simulink model "Tricopter_Controlled"  (R2015a)
settings: Solver=ode3  SolverMode=SingleTasking  StartTime=0.0  StopTime=inf  FixedStep=T_sim  RelTol=1e-3
values from neighbouring files (symbols this model uses):
  A_l_max_x = sqrt( (A_z_max)^2  -  g^2  )    [Run3Copter.m]
  A_l_max_y = g*tand(15)    [Run3Copter.m]
  A_z_max = Max_Thrust*3/m    [Run3Copter.m]
  Alt_0 = input(' Give the initial altitude (m): ')    [Run3Copter.m]
  B_hover_4dof = [-0.192641491537 -0.295051706147 -72.3190840892 -0.00308714144823 24.9504828653 -1.18743631629 9.87469464114e-05 6.48783896558 -0.0529805907426 -0.000387203135788 0.131620058452 2.24065603044 ... (54 elements, 6x9)]    [Effectiv_matrices.mat]
  CG_0 = [0,0,0.02]'    [SetupComplete.m]
  epsilon = 0.01    [Run3Copter.m]
  eta_23 = deg2rad(-1.3)    [Run3Copter.m]
  g = 9.81    [SetupComplete.m]
  h = 0.08    [SetupComplete.m]
  h_M = 0.064    [SetupComplete.m]
  Hover_eta_23 = deg2rad(-1.3)    [Run3Copter.m]
  Hover_throtle_1 = 0.745    [Run3Copter.m]
  Hover_throtle_23 = Hover_throtle_1/cos(Hover_eta_23)    [Run3Copter.m]
  I_BAC_0 = [ Ix,0,Ixz;0,Iy,0;Ixz,0,Iz]    [SetupComplete.m]
  Initial_Omegas = Omega_hover    [Run3Copter.m]
  Initial_Torques = Torque_hover    [Run3Copter.m]
  Ix = 0.103    [SetupComplete.m]
  Iy = 0.147    [SetupComplete.m]
  Iz = 0.237    [SetupComplete.m]
  l = 0.345    [SetupComplete.m]
  l_arm = 0.264    [SetupComplete.m]
  latitude = 52.071118    [Run3Copter.m]
  longitude = -0.627404    [Run3Copter.m]
  m = 3.51    [SetupComplete.m]
  m_0 = 2.61    [SetupComplete.m]
  m_M = 0.300    (= 0.3)    [SetupComplete.m]
  Rotation_sign = [ 1,-1,-1]    [SetupComplete.m]
  T_ctrl = 0.02    [Run3Copter.m]
  T_sim = 0.01    [Run3Copter.m]
  throtle_1 = 0*0.745    (= 0)    [Run3Copter.m]
  throtle_23 = throtle_1/cos(eta_23)    [Run3Copter.m]
  v_i0 = sqrt( 1/3*m*g/(2*rho*pi*R^2)  )    [SetupComplete.m]
undefined symbols (not defined in the file or in its folder): DOWN_0, EAST_0, Newton, NORTH_0, P_0, Q_0, R_0, Raphson, U_0, V_0, W_0
libraries: XXCopter_Control x64, simulink_extras x17, simulink x11, XXCopter x8
(part 4 of 6)

== system Tricopter_Controlled/TriCopter FCS/TriCopter FCS/Control and guidance/Inner PI Controller Quaternions/Attitude Controller ==
  AWU : Inport
  Phi_ref (rad) : Inport  Port=2
  q_ref : Inport  Port=3
  Yaw_ref (rad) : Inport  Port=4
  All_meas : Inport  Port=5
  activation_bus : Inport  Port=6
  init_cond : Inport  Port=7
  AWU1 : InportShadow
  AWU2 : InportShadow
  Build Pseudo_theta : MATLAB Function  TreatAsAtomicUnit=on
  Build Pseudo_theta1 : MATLAB Function  TreatAsAtomicUnit=on
  Bus Creator : BusCreator  Inputs=3
  Bus Creator1 : BusCreator  Inputs=3
  Bus Creator2 : BusCreator  Inputs=3
  Bus Selector : BusSelector  OutputSignals=Meas.Eulr_meas_rad,Meas.q_meas
  Bus Selector1 : BusSelector  OutputSignals=att_act
  Bus Selector2 : BusSelector  OutputSignals=att_init
  Bus Selector3 : BusSelector  OutputSignals=att_init
  Bus Selector4 : BusSelector  OutputSignals=att_init
  Mux : Mux  Inputs=3
  Ref Model and PI Controller : XXCopter_Control/Ref Model and PI Controller  delta=0  tau=2  RisingSlewLimit=deg2rad(8)  FallingSlewLimit=-deg2rad(8)  K_f=0  K_a=1  Con_way=pro  omega_n=4  xi=0.5  Z1=-30  K_b=2  f_i=0.15  f_c=1
  Ref Model and PI Controller1 : XXCopter_Control/Ref Model and PI Controller  delta=0  tau=1.5  RisingSlewLimit=deg2rad(8)  FallingSlewLimit=-deg2rad(8)  K_f=0  K_a=1  Con_way=pro  omega_n=4  xi=0.5  Z1=-30  K_b=1.2  f_i=0.1  f_c=1
  Ref Model and PI Controller2 : XXCopter_Control/Ref Model and PI Controller  delta=0  tau=1.5  RisingSlewLimit=deg2rad(8)  FallingSlewLimit=-deg2rad(8)  K_f=0  K_a=1  Con_way=pro  omega_n=4  xi=0.5  Z1=-30  K_b=1.5  f_i=0.1  f_c=1
  Retrieve quaternion : MATLAB Function  TreatAsAtomicUnit=on
  Selector : Selector  InputPortWidth=3
  Selector1 : Selector  InputPortWidth=3
  Selector2 : Selector  InputPortWidth=3  Indices=3
  Selector3 : Selector  InputPortWidth=3  Indices=2
  Selector4 : Selector  InputPortWidth=3  Indices=3
  Selector5 : Selector  InputPortWidth=3
  Selector6 : Selector  InputPortWidth=3  Indices=2
  Selector7 : Selector  InputPortWidth=3  Indices=3
  Sum : Sum  Inputs=+-|
  Sum1 : Sum  Inputs=+-|
  Sum2 : Sum  Inputs=+-|
  Terminator1 : Terminator
  Terminator2 : Terminator
  Terminator3 : Terminator
  Trigonometric Function : Trigonometry
  init_cond1 : InportShadow  Port=7
  init_cond2 : InportShadow  Port=7
  quat_dot des (rad/s) : Outport
  wires:
  Ref Model and PI Controller/4 -> Sum2/2
  Sum2/1 -> Bus Creator2/3  "Vz_err"
  Ref Model and PI Controller/3 -> Bus Creator2/2, Sum2/1  "Vz_sf"
  Ref Model and PI Controller/2 -> Bus Creator2/1  "Vz_sf_dot"
  Ref Model and PI Controller1/4 -> Sum1/2
  Sum1/1 -> Bus Creator1/3  "Vy_err"
  Ref Model and PI Controller1/3 -> Bus Creator1/2, Sum1/1  "Vy_sf"
  Ref Model and PI Controller1/2 -> Bus Creator1/1  "Vy_sf_dot"
  Ref Model and PI Controller2/4 -> Sum/2
  Bus Creator2/1 -> Terminator3/1
  Bus Creator1/1 -> Terminator1/1
  Bus Creator/1 -> Terminator2/1
  Sum/1 -> Bus Creator/3  "Vx_err"
  Ref Model and PI Controller2/3 -> Bus Creator/2, Sum/1  "Vx_sf"
  Ref Model and PI Controller2/2 -> Bus Creator/1  "Vx_sf_dot"
  Yaw_ref (rad)/1 -> Ref Model and PI Controller/1
  Selector/1 -> Ref Model and PI Controller2/2
  Bus Selector/2 -> Retrieve quaternion/2(q), Build Pseudo_theta1/1(q)  "<q_meas>"
  All_meas/1 -> Bus Selector/1
  q_ref/1 -> Build Pseudo_theta/1(q)
  Phi_ref (rad)/1 -> Ref Model and PI Controller2/1
  Retrieve quaternion/1(qdot) -> quat_dot des (rad/s)/1
  Ref Model and PI Controller2/1 -> Mux/1
  Ref Model and PI Controller/1 -> Mux/3
  Ref Model and PI Controller1/1 -> Mux/2
  Mux/1 -> Retrieve quaternion/1(Pseudoeuler_dot)
  Selector2/1 -> Ref Model and PI Controller/2
  Bus Selector/1 -> Selector2/1, Selector/1  "<Eulr_meas_rad>"
  Build Pseudo_theta1/1(Pseudo_theta) -> Ref Model and PI Controller1/2
  Build Pseudo_theta/1(Pseudo_theta) -> Ref Model and PI Controller1/1
  AWU/1 -> Selector1/1
  AWU1/1 -> Selector3/1
  AWU2/1 -> Selector4/1
  Selector3/1 -> Trigonometric Function/1
  Selector1/1 -> Ref Model and PI Controller2/4
  Trigonometric Function/1 -> Ref Model and PI Controller1/4
  Selector4/1 -> Ref Model and PI Controller/4
  activation_bus/1 -> Bus Selector1/1
  Bus Selector1/1 -> Ref Model and PI Controller/Enable, Ref Model and PI Controller1/Enable, Ref Model and PI Controller2/Enable  "<att_act>"
  init_cond/1 -> Bus Selector2/1
  Bus Selector2/1 -> Selector5/1  "<att_init>"
  Selector5/1 -> Ref Model and PI Controller2/3
  Selector6/1 -> Ref Model and PI Controller1/3
  init_cond1/1 -> Bus Selector3/1
  Bus Selector3/1 -> Selector6/1  "<att_init>"
  init_cond2/1 -> Bus Selector4/1
  Selector7/1 -> Ref Model and PI Controller/3
  Bus Selector4/1 -> Selector7/1  "<att_init>"

== system Tricopter_Controlled/TriCopter FCS/TriCopter FCS/Control and guidance/Inner PI Controller Quaternions/Body Rates Controller ==
  p_ref : Inport
  q_ref : Inport  Port=2
  r_ref : Inport  Port=3
  All_meas : Inport  Port=4
  init_cond : Inport  Port=5
  activation_bus : Inport  Port=6
  Bus Creator : BusCreator
  Bus Creator1 : BusCreator
  Bus Creator2 : BusCreator
  Bus Selector : BusSelector  OutputSignals=Meas.omega_b_meas_radps
  Bus Selector1 : BusSelector  OutputSignals=omega_b_act
  Bus Selector2 : BusSelector  OutputSignals=b_rates_init
  Bus Selector3 : BusSelector  OutputSignals=b_rates_init
  Bus Selector4 : BusSelector  OutputSignals=b_rates_init
  Mux : Mux  Inputs=3
  Ref Model and P Controller p : XXCopter_Control/Ref Model and P Controller  tau=0.7  RisingSlewLimit=4  FallingSlewLimit=-4  K_f=0.7  K_b=6
  Ref Model and P Controller q : XXCopter_Control/Ref Model and P Controller  tau=0.7  RisingSlewLimit=4  FallingSlewLimit=-4  K_f=0.7  K_b=6
  Ref Model and P Controller r : XXCopter_Control/Ref Model and P Controller  tau=1.5  RisingSlewLimit=4  FallingSlewLimit=-4  K_f=0.7  K_b=1.5
  Selector : Selector  InputPortWidth=3
  Selector1 : Selector  InputPortWidth=3  Indices=2
  Selector2 : Selector  InputPortWidth=3  Indices=3
  Selector3 : Selector  InputPortWidth=3
  Selector4 : Selector  InputPortWidth=3  Indices=2
  Selector5 : Selector  InputPortWidth=3  Indices=3
  Sum : Sum  Inputs=+-|
  Sum1 : Sum  Inputs=+-|
  Sum2 : Sum  Inputs=+-|
  Terminator1 : Terminator
  Terminator2 : Terminator
  Terminator3 : Terminator
  init_cond1 : InportShadow  Port=5
  init_cond2 : InportShadow  Port=5
  Angular acc des (rad/s^2) : Outport
  wires:
  Ref Model and P Controller r/5 -> Bus Creator2/4  "K_b_r"
  Ref Model and P Controller r/4 -> Sum2/2
  Sum2/1 -> Bus Creator2/3  "r_err"
  Ref Model and P Controller r/3 -> Bus Creator2/2, Sum2/1  "r_sf"
  Ref Model and P Controller r/2 -> Bus Creator2/1  "r_sf_dot"
  Ref Model and P Controller q/5 -> Bus Creator1/4  "K_b_q"
  Ref Model and P Controller q/4 -> Sum1/2
  Sum1/1 -> Bus Creator1/3  "q_err"
  Ref Model and P Controller q/3 -> Bus Creator1/2, Sum1/1  "q_sf"
  Ref Model and P Controller q/2 -> Bus Creator1/1  "q_sf_dot"
  Ref Model and P Controller p/5 -> Bus Creator/4  "K_b_p"
  Ref Model and P Controller p/4 -> Sum/2
  Selector2/1 -> Ref Model and P Controller r/2
  Bus Creator2/1 -> Terminator3/1
  Bus Creator1/1 -> Terminator1/1
  Bus Creator/1 -> Terminator2/1
  Sum/1 -> Bus Creator/3  "p_err"
  Ref Model and P Controller p/3 -> Bus Creator/2, Sum/1  "p_sf"
  Ref Model and P Controller p/2 -> Bus Creator/1  "p_sf_dot"
  r_ref/1 -> Ref Model and P Controller r/1
  Selector1/1 -> Ref Model and P Controller q/2
  q_ref/1 -> Ref Model and P Controller q/1
  Mux/1 -> Angular acc des (rad/s^2)/1
  p_ref/1 -> Ref Model and P Controller p/1
  Bus Selector/1 -> Selector2/1, Selector/1, Selector1/1  "<omega_b_meas_radps>"
  All_meas/1 -> Bus Selector/1
  Ref Model and P Controller r/1 -> Mux/3
  Ref Model and P Controller q/1 -> Mux/2
  Ref Model and P Controller p/1 -> Mux/1
  Selector/1 -> Ref Model and P Controller p/2
  activation_bus/1 -> Bus Selector1/1
  Bus Selector1/1 -> Ref Model and P Controller p/Enable, Ref Model and P Controller r/Enable, Ref Model and P Controller q/Enable  "<omega_b_act>"
  init_cond/1 -> Bus Selector2/1
  Bus Selector2/1 -> Selector3/1  "<b_rates_init>"
  Selector3/1 -> Ref Model and P Controller p/3
  init_cond1/1 -> Bus Selector3/1
  Bus Selector3/1 -> Selector4/1  "<b_rates_init>"
  Selector4/1 -> Ref Model and P Controller q/3
  init_cond2/1 -> Bus Selector4/1
  Bus Selector4/1 -> Selector5/1  "<b_rates_init>"
  Selector5/1 -> Ref Model and P Controller r/3

== system Tricopter_Controlled/TriCopter FCS/TriCopter FCS/Control and guidance/Inner PI Controller Quaternions/Limits in Ang accel ==
  note: Here it is assumed that at all time every prop is generating m*g/3 newtons of force . It is conservative?
  Ang Ace des : Inport
  Euler meas : Inport  Port=2
  Limis eval : MATLAB Function  TreatAsAtomicUnit=on
  Saturation Dynamic : simulink/Discontinuities/Saturation Dynamic  OutMin=[]  OutMax=[]  OutDataTypeStr=Inherit: Same as second input  OutDataType=fixdt(1, 16)  OutScaling=2^-10  DoSatur=off
  ang Ace des : Outport
  wires:
  Limis eval/1(Limit_up) -> Saturation Dynamic/1
  Limis eval/2(Limit_down) -> Saturation Dynamic/3
  Euler meas/1 -> Limis eval/2(euler_ang)
  Ang Ace des/1 -> Saturation Dynamic/2, Limis eval/1(Ang_Accel)
  Saturation Dynamic/1 -> ang Ace des/1

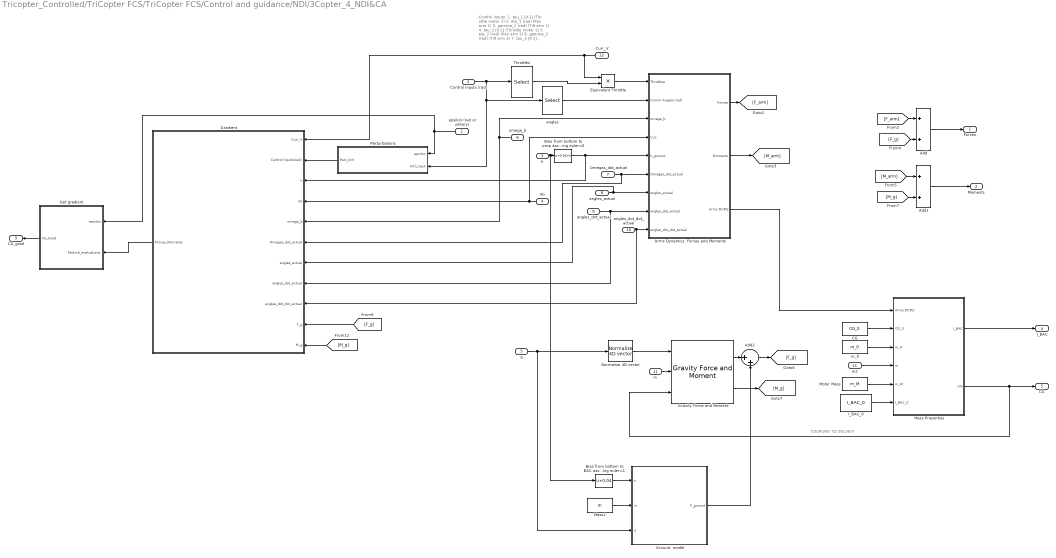
== system Tricopter_Controlled/TriCopter FCS/TriCopter FCS/Control and guidance/NDI/3Copter_4_NDI&CA ==
  note: Control inputs:
      | 1. tau_1 [0-1] (Thr ottle motor 1)
      | 2. eta_1 (rad)  (Pan arm 1)
      | 3. gamma_1 (rad)  (Tilt arm 1)
      |
      | 4. tau_2 [0-1] (Throttle motor 2)
      | 5. eta_2 (rad)  (Pan arm 2)
      | 6. gamma_2 (rad)  (Tilt arm 2)
      |
      | 7. tau_3 [0-1] (Throttle motor 3)
      | 8. eta_3 (rad)  (Pan arm  3)
      | 9. gamma_3 (rad)  (Tilt arm 3)
  note: COUPLING TO SOLVE!!!
  "epsilon (rad or unitary) " : Inport
  Control Inputs (rad) : Inport  Port=2
  h : Inport  Port=3
  Vb : Inport  Port=4
  q : Inport  Port=5
  omega_b : Inport  Port=6
  Omegas_dot_actual : Inport  Port=7
  angles_actual : Inport  Port=8
  angles_dot_actual : Inport  Port=9
  angles_dot_dot_actual : Inport  Port=10
  " m" : Inport  Port=11
  Curr_V : Inport  Port=12
  Add : Sum
  Add1 : Sum
  Add2 : Sum  Inputs=|++
  Arms Dynamics: Forces and Moments : Subsystem  TreatAsAtomicUnit=on
  Bias from bottom to BAC assuming euler=1 : Bias  Bias=0.04
  Bias from bottom to prop assuming euler=0 : Bias  Bias=0.04+h
  CG : Constant  Value=CG_0
  Equivalent Throttle : Product  Inputs=**
  Get gradient : MATLAB Function  TreatAsAtomicUnit=on
  Gradient : Subsystem  TreatAsAtomicUnit=on
  Gravity Force and Moment : XXCopter_Control/Gravity Force and Moment
  Ground  model : Subsystem  TreatAsAtomicUnit=on
  I_BAC_0 : Constant  Value=I_BAC_0
  Mass Properties : Subsystem  TreatAsAtomicUnit=on
  Mass2 : Constant  Value=m
  Motor Mass : Constant  Value=m_M
  Normalize 4D vector : XXCopter/Normalize 4D vector
  Perturbations : MATLAB Function  TreatAsAtomicUnit=on
  Throttles : Selector  IndexMode=Zero-based  InputPortWidth=9  Indices=[0,3,6]
  "angles " : Selector  IndexMode=Zero-based  InputPortWidth=9  Indices=[1,2,4,5,7,8]
  m2 : InportShadow  Port=11
  m_0 : Constant  Value=m_0
  Forces : Outport
  Moments : Outport  Port=2
  CA_grad : Outport  Port=3
  I_BAC : Outport  Port=4
  "CG " : Outport  Port=5
  wires:
  Get gradient/1(CA_Grad) -> CA_grad/1
  "epsilon (rad or unitary) "/1 -> Perturbations/1(epsilon), Get gradient/1(epsilon)
  Perturbations/1(Pert_Ctrl) -> Gradient/2("Control Inputs(rad) ")
  Gradient/1(Forces_Moments) -> Get gradient/2(Perturb_evaluations)
  Mass Properties/1(I_BAC) -> I_BAC/1
  [F_g] -> Gradient/10(F_g)
  [M_g] -> Gradient/11(M_g)
  Normalize 4D vector/1 -> Gravity Force and Moment/1
  angles_dot_actual/1 -> Arms Dynamics: Forces and Moments/8(angles_dot_actual), Gradient/8(angles_dot_actual)
  Omegas_dot_actual/1 -> Gradient/6(Omegas_dot_actual), Arms Dynamics: Forces and Moments/6(Omegas_dot_actual)
  Add1/1 -> Moments/1
  Curr_V/1 -> Gradient/1(Curr_V), Equivalent Throttle/1
  Equivalent Throttle/1 -> Arms Dynamics: Forces and Moments/1(Throttles)
  Mass Properties/2(CG) -> Gravity Force and Moment/3, "CG "/1
  Add/1 -> Forces/1
  m2/1 -> Mass Properties/4(m)
  m_0/1 -> Mass Properties/3(m_0)
  I_BAC_0/1 -> Mass Properties/6(I_BAC_0)
  Motor Mass/1 -> Mass Properties/5(m_M)
  CG/1 -> Mass Properties/2(CG_0)
  Arms Dynamics: Forces and Moments/3(Arms DCMs) -> Mass Properties/1(Arms DCMs)
  Control Inputs (rad)/1 -> Throttles/1, Perturbations/2(Ctrl_input), "angles "/1
  Throttles/1 -> Equivalent Throttle/2
  [M_g] -> Add1/2
  [M_arm] -> Add1/1
  [F_g] -> Add/2
  [F_arm] -> Add/1
  Gravity Force and Moment/2 -> [M_g]
  Arms Dynamics: Forces and Moments/2(Moments) -> [M_arm]
  Arms Dynamics: Forces and Moments/1(Forces) -> [F_arm]
  " m"/1 -> Gravity Force and Moment/2
  omega_b/1 -> Gradient/5(omega_b), Arms Dynamics: Forces and Moments/3(omega_b)
  Vb/1 -> Arms Dynamics: Forces and Moments/4(V_b), Gradient/4(Vb)
  angles_actual/1 -> Gradient/7(angles_actual), Arms Dynamics: Forces and Moments/7(angles_actual)
  "angles "/1 -> Arms Dynamics: Forces and Moments/2(Comm Angles (rad))
  angles_dot_dot_actual/1 -> Gradient/9(angles_dot_dot_actual), Arms Dynamics: Forces and Moments/9(angles_dot_dot_actual)
  Bias from bottom to prop assuming euler=0/1 -> Arms Dynamics: Forces and Moments/5(h_ground), Gradient/3(h)
  Ground  model/1(F_ground) -> Add2/2
  q/1 -> Normalize 4D vector/1, Ground  model/3(q)
  Mass2/1 -> Ground  model/2(m)
  Bias from bottom to BAC assuming euler=1/1 -> Ground  model/1(h)
  h/1 -> Bias from bottom to prop assuming euler=0/1, Bias from bottom to BAC assuming euler=1/1
  Gravity Force and Moment/1 -> Add2/1
  Add2/1 -> [F_g]

== system Tricopter_Controlled/TriCopter FCS/TriCopter FCS/Control and guidance/Otter Overactuated P Controller/Position Controller ==
  AWU : Inport
  X_e_x_ref : Inport  Port=2
  X_e_y_ref : Inport  Port=3
  X_e_z_ref : Inport  Port=4
  activation_bus : Inport  Port=5
  All_meas : Inport  Port=6
  init_cond : Inport  Port=7
  AWU1 : InportShadow
  AWU2 : InportShadow
  Bus Creator : BusCreator  Inputs=3
  Bus Creator1 : BusCreator  Inputs=3
  Bus Creator2 : BusCreator  Inputs=3
  Bus Selector : BusSelector  OutputSignals=Meas.Pos_meas_m
  Bus Selector1 : BusSelector  OutputSignals=pos_xy_init
  Bus Selector2 : BusSelector  OutputSignals=pos_xy_act
  Bus Selector3 : BusSelector  OutputSignals=alt_init
  Bus Selector4 : BusSelector  OutputSignals=alt_act
  Mux : Mux  Inputs=3
  Ref Model and PI Controller : XXCopter_Control/Ref Model and PI Controller  delta=0  tau=3  RisingSlewLimit=4  FallingSlewLimit=-4  K_f=0  K_a=1  Con_way=pro  omega_n=4  xi=0.5  Z1=-30  K_b=1.2  f_i=0.07  f_c=1
  Ref Model and PI Controller1 : XXCopter_Control/Ref Model and PI Controller  delta=0  tau=5  RisingSlewLimit=4  FallingSlewLimit=-4  K_f=0  K_a=1  Con_way=pro  omega_n=4  xi=0.5  Z1=-30  K_b=1  f_i=0.07  f_c=1
  Ref Model and PI Controller3 : XXCopter_Control/Ref Model and PI Controller  delta=0  tau=5  RisingSlewLimit=4  FallingSlewLimit=-4  K_f=0  K_a=1  Con_way=pro  omega_n=4  xi=0.5  Z1=-30  K_b=1  f_i=0.07  f_c=1
  Selector : Selector  InputPortWidth=3
  Selector1 : Selector  InputPortWidth=3  Indices=2
  Selector2 : Selector  InputPortWidth=3  Indices=3
  Selector3 : Selector  InputPortWidth=3
  Selector4 : Selector  InputPortWidth=3  Indices=2
  Selector5 : Selector  InputPortWidth=3  Indices=3
  Selector6 : Selector  InputPortWidth=2
  Selector7 : Selector  InputPortWidth=2  Indices=2
  Sum : Sum  Inputs=+-|
  Sum1 : Sum  Inputs=+-|
  Sum2 : Sum  Inputs=+-|
  Terminator1 : Terminator
  Terminator2 : Terminator
  Terminator3 : Terminator
  Ve des (m/s) : Outport
  wires:
  All_meas/1 -> Bus Selector/1
  Bus Selector/1 -> Selector/1, Selector1/1, Selector2/1  "<Pos_meas_m>"
  X_e_x_ref/1 -> Ref Model and PI Controller3/1
  Ref Model and PI Controller3/1 -> Mux/1
  Mux/1 -> Ve des (m/s)/1
  X_e_y_ref/1 -> Ref Model and PI Controller1/1
  X_e_z_ref/1 -> Ref Model and PI Controller/1
  Ref Model and PI Controller1/1 -> Mux/2
  Ref Model and PI Controller/1 -> Mux/3
  Ref Model and PI Controller3/2 -> Bus Creator/1  "X_ex_sf_dot"
  Ref Model and PI Controller3/3 -> Bus Creator/2, Sum/1  "X_ex_sf"
  Sum/1 -> Bus Creator/3  "X_ex_err"
  Bus Creator/1 -> Terminator2/1
  Bus Creator1/1 -> Terminator1/1
  Bus Creator2/1 -> Terminator3/1
  Ref Model and PI Controller3/4 -> Sum/2
  Ref Model and PI Controller1/2 -> Bus Creator1/1  "X_ey_sf_dot"
  Ref Model and PI Controller1/3 -> Sum1/1, Bus Creator1/2  "X_e_y_sf"
  Sum1/1 -> Bus Creator1/3  "X_ey_err"
  Ref Model and PI Controller1/4 -> Sum1/2
  Ref Model and PI Controller/2 -> Bus Creator2/1  "X_ez_sf_dot"
  Ref Model and PI Controller/3 -> Sum2/1, Bus Creator2/2  "X_ez_sf"
  Sum2/1 -> Bus Creator2/3  "X_ez_err"
  Ref Model and PI Controller/4 -> Sum2/2
  AWU/1 -> Selector3/1
  AWU1/1 -> Selector4/1
  AWU2/1 -> Selector5/1
  Selector3/1 -> Ref Model and PI Controller3/4
  Selector4/1 -> Ref Model and PI Controller1/4
  Selector5/1 -> Ref Model and PI Controller/4
  Selector2/1 -> Ref Model and PI Controller/2
  Selector1/1 -> Ref Model and PI Controller1/2
  Selector/1 -> Ref Model and PI Controller3/2
  init_cond/1 -> Bus Selector1/1, Bus Selector3/1
  activation_bus/1 -> Bus Selector4/1, Bus Selector2/1
  Bus Selector2/1 -> Ref Model and PI Controller1/Enable, Ref Model and PI Controller3/Enable  "<pos_xy_act>"
  Bus Selector1/1 -> Selector7/1, Selector6/1  "<pos_xy_init>"
  Selector6/1 -> Ref Model and PI Controller3/3
  Selector7/1 -> Ref Model and PI Controller1/3
  Bus Selector3/1 -> Ref Model and PI Controller/3  "<alt_init>"
  Bus Selector4/1 -> Ref Model and PI Controller/Enable  "<alt_act>"

== system Tricopter_Controlled/TriCopter FCS/TriCopter FCS/Control and guidance/Otter Overactuated P Controller/Velocity Controller ==
  Vyaw_x_ref : Inport
  Vyaw_y_ref : Inport  Port=2
  Vyaw_z_ref : Inport  Port=3
  V_yaw_meas : Inport  Port=4
  activation_bus : Inport  Port=5
  Init_cond : Inport  Port=6
  Bus Creator : BusCreator
  Bus Creator1 : BusCreator
  Bus Creator2 : BusCreator
  Bus Selector1 : BusSelector  OutputSignals=vel_yaw_z_act
  Bus Selector2 : BusSelector  OutputSignals=vel_yaw_xy_act
  Bus Selector3 : BusSelector  OutputSignals=vel_yaw_xy_init
  Bus Selector4 : BusSelector  OutputSignals=vel_yaw_z_init
  Mux : Mux  Inputs=3
  Ref Model and P Controller p : XXCopter_Control/Ref Model and P Controller  tau=2  RisingSlewLimit=1  FallingSlewLimit=-1  K_f=0.5  K_b=1
  Ref Model and P Controller q : XXCopter_Control/Ref Model and P Controller  tau=2  RisingSlewLimit=1  FallingSlewLimit=-1  K_f=0.5  K_b=1
  Ref Model and P Controller r : XXCopter_Control/Ref Model and P Controller  tau=1  RisingSlewLimit=1  FallingSlewLimit=-1  K_f=0.4  K_b=8
  Selector : Selector  InputPortWidth=3
  Selector1 : Selector  InputPortWidth=3  Indices=2
  Selector2 : Selector  InputPortWidth=3  Indices=3
  Selector3 : Selector  InputPortWidth=2
  Selector4 : Selector  InputPortWidth=2  Indices=2
  Sum : Sum  Inputs=+-|
  Sum1 : Sum  Inputs=+-|
  Sum2 : Sum  Inputs=+-|
  Terminator1 : Terminator
  Terminator2 : Terminator
  Terminator3 : Terminator
  Acc_yaw des (m/s) : Outport
  wires:
  Ref Model and P Controller r/5 -> Bus Creator2/4  "K_b_Ve_z"
  Ref Model and P Controller r/4 -> Sum2/2
  Sum2/1 -> Bus Creator2/3  "Vez_err"
  Ref Model and P Controller r/3 -> Bus Creator2/2, Sum2/1  "Vez_sf"
  Ref Model and P Controller r/2 -> Bus Creator2/1  "Vez_sf_dot"
  Ref Model and P Controller q/5 -> Bus Creator1/4  "K_b_Vey"
  Ref Model and P Controller q/4 -> Sum1/2
  Sum1/1 -> Bus Creator1/3  "Vey_err"
  Ref Model and P Controller q/3 -> Bus Creator1/2, Sum1/1  "Ve_y_sf"
  Ref Model and P Controller q/2 -> Bus Creator1/1  "Vey_sf_dot"
  Ref Model and P Controller p/5 -> Bus Creator/4  "K_b_Vex"
  Ref Model and P Controller p/4 -> Sum/2
  Selector2/1 -> Ref Model and P Controller r/2
  Bus Creator2/1 -> Terminator3/1
  Bus Creator1/1 -> Terminator1/1
  Bus Creator/1 -> Terminator2/1
  Sum/1 -> Bus Creator/3  "Vex_err"
  Ref Model and P Controller p/3 -> Bus Creator/2, Sum/1  "Vex_sf"
  Ref Model and P Controller p/2 -> Bus Creator/1  "Vex_sf_dot"
  Ref Model and P Controller r/1 -> Mux/3
  Ref Model and P Controller q/1 -> Mux/2
  Vyaw_z_ref/1 -> Ref Model and P Controller r/1
  Selector1/1 -> Ref Model and P Controller q/2
  Vyaw_y_ref/1 -> Ref Model and P Controller q/1
  Mux/1 -> Acc_yaw des (m/s)/1
  Ref Model and P Controller p/1 -> Mux/1
  Vyaw_x_ref/1 -> Ref Model and P Controller p/1
  V_yaw_meas/1 -> Selector1/1, Selector/1, Selector2/1
  Selector/1 -> Ref Model and P Controller p/2
  activation_bus/1 -> Bus Selector1/1, Bus Selector2/1
  Bus Selector2/1 -> Ref Model and P Controller q/Enable, Ref Model and P Controller p/Enable  "<vel_yaw_xy_act>"
  Bus Selector1/1 -> Ref Model and P Controller r/Enable  "<vel_yaw_z_act>"
  Init_cond/1 -> Bus Selector4/1, Bus Selector3/1
  Bus Selector3/1 -> Selector3/1, Selector4/1  "<vel_yaw_xy_init>"
  Selector3/1 -> Ref Model and P Controller p/3
  Selector4/1 -> Ref Model and P Controller q/3
  Bus Selector4/1 -> Ref Model and P Controller r/3  "<vel_yaw_z_init>"

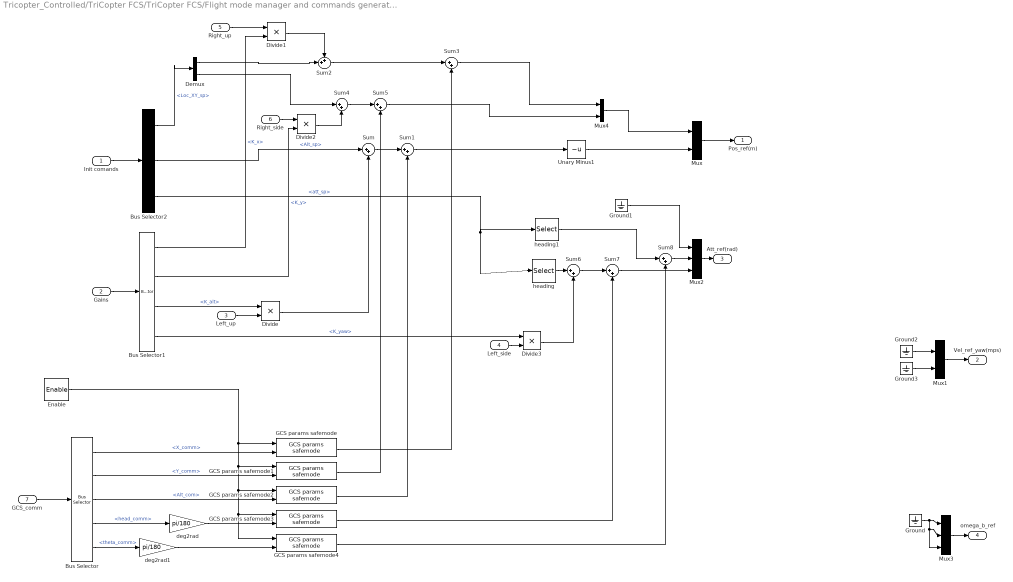
== system Tricopter_Controlled/TriCopter FCS/TriCopter FCS/Flight mode manager and commands generator/Commands generator/Full auto ==
  Init comands : Inport
  Gains : Inport  Port=2
  Left_up : Inport  Port=3
  Left_side : Inport  Port=4
  Right_up : Inport  Port=5
  Right_side : Inport  Port=6
  GCS_comm : Inport  Port=7
  Enable : EnablePort  StatesWhenEnabling=reset  ShowOutputPort=on
  Bus Selector : BusSelector  OutputSignals=X_comm,Y_comm,Alt_com,head_comm,theta_comm
  Bus Selector1 : BusSelector  OutputSignals=K_x,K_y,K_alt,K_yaw
  Bus Selector2 : BusSelector  OutputSignals=Loc_XY_sp,Alt_sp,att_sp
  Demux : Demux  Outputs=2
  Divide{,1..3} (4 alike) : Product  Inputs=**
  GCS params safemode{,1..4} (5 alike) : XXCopter_Control/GCS params safemode
  Ground{,1..3} (4 alike) : Ground
  Mux : Mux  Inputs=[2,1]
  Mux1 : Mux  Inputs=[2,1]
  Mux2 : Mux  Inputs=3
  Mux3 : Mux  Inputs=3
  Mux4 : Mux  Inputs=2
  Sum{,1,3..8} (8 alike) : Sum  Inputs=|++
  Sum2 : Sum  Inputs=++|
  Unary Minus1 : UnaryMinus
  deg2rad : Gain  Gain=pi/180
  deg2rad1 : Gain  Gain=pi/180
  heading : Selector  InputPortWidth=3  Indices=3
  heading1 : Selector  InputPortWidth=3  Indices=2
  Pos_ref(m) : Outport
  Vel_ref_yaw(mps) : Outport  Port=2
  Att_ref(rad) : Outport  Port=3
  omega_b_ref : Outport  Port=4
  wires:
  Bus Selector2/2 -> Sum/1  "<Alt_sp>"
  Divide/1 -> Sum/2
  Sum/1 -> Sum1/1
  GCS params safemode2/1 -> Sum1/2
  Sum1/1 -> Unary Minus1/1
  GCS_comm/1 -> Bus Selector/1
  Bus Selector/1 -> GCS params safemode/2  "<X_comm>"
  Bus Selector/2 -> GCS params safemode1/2  "<Y_comm>"
  Bus Selector/3 -> GCS params safemode2/2  "<Alt_com>"
  Bus Selector/4 -> deg2rad/1  "<head_comm>"
  Mux1/1 -> Vel_ref_yaw(mps)/1
  Mux/1 -> Pos_ref(m)/1
  Mux2/1 -> Att_ref(rad)/1
  Unary Minus1/1 -> Mux/2
  Ground/1 -> Mux3/3, Mux3/2, Mux3/1
  Ground1/1 -> Mux2/1
  Ground2/1 -> Mux1/1
  Ground3/1 -> Mux1/2
  Mux4/1 -> Mux/1
  Mux3/1 -> omega_b_ref/1
  Gains/1 -> Bus Selector1/1
  Init comands/1 -> Bus Selector2/1
  Bus Selector1/3 -> Divide/1  "<K_alt>"
  Left_up/1 -> Divide/2
  Bus Selector2/1 -> Demux/1  "<Loc_XY_sp>"
  Sum2/1 -> Sum3/1
  Sum3/1 -> Mux4/1
  GCS params safemode/1 -> Sum3/2
  Demux/1 -> Sum2/2
  Right_up/1 -> Divide1/1
  Bus Selector1/1 -> Divide1/2  "<K_x>"
  Divide1/1 -> Sum2/1
  Sum4/1 -> Sum5/1
  GCS params safemode1/1 -> Sum5/2
  Sum5/1 -> Mux4/2
  Divide2/1 -> Sum4/2
  Demux/2 -> Sum4/1
  Right_side/1 -> Divide2/1
  Bus Selector1/2 -> Divide2/2  "<K_y>"
  Sum6/1 -> Sum7/1
  Sum7/1 -> Mux2/3
  GCS params safemode3/1 -> Sum7/2
  heading/1 -> Sum6/1
  Bus Selector2/3 -> heading1/1, heading/1  "<att_sp>"
  Bus Selector1/4 -> Divide3/1  "<K_yaw>"
  Left_side/1 -> Divide3/2
  Divide3/1 -> Sum6/2
  Bus Selector/5 -> deg2rad1/1  "<theta_comm>"
  GCS params safemode4/1 -> Sum8/2
  heading1/1 -> Sum8/1
  Sum8/1 -> Mux2/2
  deg2rad/1 -> GCS params safemode3/2
  deg2rad1/1 -> GCS params safemode4/2
  Enable/1 -> GCS params safemode4/1, GCS params safemode3/1, GCS params safemode2/1, GCS params safemode1/1, GCS params safemode/1

== system Tricopter_Controlled/TriCopter FCS/TriCopter FCS/Flight mode manager and commands generator/Commands generator/Home ==
  Init comands : Inport
  Gains : Inport  Port=2
  Left_up : Inport  Port=3
  Left_side : Inport  Port=4
  Right_up : Inport  Port=5
  Right_side : Inport  Port=6
  GCS_comm : Inport  Port=7
  Enable : EnablePort  StatesWhenEnabling=reset
  Bus Selector2 : BusSelector  OutputSignals=Loc_XY_sp,Alt_sp,att_sp
  Ground{,1..3} (4 alike) : Ground
  Mux : Mux  Inputs=[2,1]
  Mux1 : Mux  Inputs=[2,1]
  Mux2 : Mux  Inputs=3
  Selector : Selector  InputPortWidth=3  Indices=3
  Terminator{,1..5} (6 alike) : Terminator
  Unary Minus : UnaryMinus
  Pos_ref(m) : Outport
  Vel_ref_yaw(mps) : Outport  Port=2
  Att_ref(rad) : Outport  Port=3
  omega_b_ref : Outport  Port=4
  wires:
  Mux1/1 -> Vel_ref_yaw(mps)/1
  Mux2/1 -> Att_ref(rad)/1
  Ground1/1 -> Mux2/2, Mux2/1
  Ground2/1 -> Mux1/1
  Ground3/1 -> Mux1/2
  Mux/1 -> Pos_ref(m)/1
  Ground/1 -> omega_b_ref/1
  Gains/1 -> Terminator/1
  Right_up/1 -> Terminator1/1
  Left_up/1 -> Terminator2/1
  Left_side/1 -> Terminator3/1
  Right_side/1 -> Terminator4/1
  GCS_comm/1 -> Terminator5/1
  Init comands/1 -> Bus Selector2/1
  Bus Selector2/1 -> Mux/1  "<Loc_XY_sp>"
  Bus Selector2/2 -> Unary Minus/1  "<Alt_sp>"
  Unary Minus/1 -> Mux/2
  Selector/1 -> Mux2/3
  Bus Selector2/3 -> Selector/1  "<att_sp>"

== system Tricopter_Controlled/TriCopter FCS/TriCopter FCS/Flight mode manager and commands generator/Commands generator/Land  ==
  Init comands : Inport
  Gains : Inport  Port=2
  Left_up : Inport  Port=3
  Left_side : Inport  Port=4
  Right_up : Inport  Port=5
  Right_side : Inport  Port=6
  GCS_comm : Inport  Port=7
  Enable : EnablePort  StatesWhenEnabling=reset
  Bus Selector2 : BusSelector  OutputSignals=Loc_XY_sp,Alt_sp,att_sp
  Ground{,1..3} (4 alike) : Ground
  Mux : Mux  Inputs=[2,1]
  Mux1 : Mux  Inputs=[2,1]
  Mux2 : Mux  Inputs=3
  Selector : Selector  InputPortWidth=3  Indices=3
  Terminator{,1..5} (6 alike) : Terminator
  Unary Minus : UnaryMinus
  Pos_ref(m) : Outport
  Vel_ref_yaw(mps) : Outport  Port=2
  Att_ref(rad) : Outport  Port=3
  omega_b_ref : Outport  Port=4
  wires:
  Mux1/1 -> Vel_ref_yaw(mps)/1
  Mux2/1 -> Att_ref(rad)/1
  Ground/1 -> omega_b_ref/1
  Ground1/1 -> Mux2/2, Mux2/1
  Ground2/1 -> Mux1/1
  Ground3/1 -> Mux1/2
  Mux/1 -> Pos_ref(m)/1
  Gains/1 -> Terminator/1
  Right_up/1 -> Terminator1/1
  Left_up/1 -> Terminator2/1
  Left_side/1 -> Terminator3/1
  Right_side/1 -> Terminator4/1
  GCS_comm/1 -> Terminator5/1
  Init comands/1 -> Bus Selector2/1
  Bus Selector2/1 -> Mux/1  "<Loc_XY_sp>"
  Bus Selector2/2 -> Unary Minus/1  "<Alt_sp>"
  Unary Minus/1 -> Mux/2
  Selector/1 -> Mux2/3
  Bus Selector2/3 -> Selector/1  "<att_sp>"

== system Tricopter_Controlled/TriCopter FCS/TriCopter FCS/Flight mode manager and commands generator/Commands generator/Man_ctrl ==
  Init comands : Inport
  Gains : Inport  Port=2
  Left_up : Inport  Port=3
  Left_side : Inport  Port=4
  Right_up : Inport  Port=5
  Right_side : Inport  Port=6
  GCS_comm : Inport  Port=7
  Enable : EnablePort  StatesWhenEnabling=reset
  Bus Selector1 : BusSelector  OutputSignals=K_vz,K_p,K_q,K_r
  Divide{1..4} (4 alike) : Product  Inputs=**
  Ground{1..2,4..5} (4 alike) : Ground
  Mux : Mux  Inputs=[2,1]
  Mux1 : Mux  Inputs=[2,1]
  Mux2 : Mux  Inputs=3
  Mux3 : Mux  Inputs=3
  Terminator : Terminator
  Terminator1 : Terminator
  Unary Minus : UnaryMinus
  Unary Minus1 : UnaryMinus
  Pos_ref(m) : Outport
  Vel_ref_yaw(mps) : Outport  Port=2
  Att_ref(rad) : Outport  Port=3
  omega_b_ref : Outport  Port=4
  wires:
  Mux1/1 -> Vel_ref_yaw(mps)/1
  Mux2/1 -> Att_ref(rad)/1
  Ground5/1 -> Mux/2
  Ground1/1 -> Mux2/3, Mux2/2, Mux2/1
  Ground2/1 -> Mux1/1
  Unary Minus1/1 -> Mux1/2
  Mux/1 -> Pos_ref(m)/1
  Mux3/1 -> omega_b_ref/1
  GCS_comm/1 -> Terminator/1
  Init comands/1 -> Terminator1/1
  Gains/1 -> Bus Selector1/1
  Bus Selector1/1 -> Divide1/2  "<K_vz>"
  Left_up/1 -> Divide1/1
  Ground4/1 -> Mux/1
  Bus Selector1/2 -> Divide2/1  "<K_p>"
  Right_side/1 -> Divide2/2
  Bus Selector1/3 -> Divide3/1  "<K_q>"
  Right_up/1 -> Divide3/2
  Bus Selector1/4 -> Divide4/1  "<K_r>"
  Left_side/1 -> Divide4/2
  Divide3/1 -> Unary Minus/1
  Divide2/1 -> Mux3/1
  Unary Minus/1 -> Mux3/2
  Divide4/1 -> Mux3/3
  Divide1/1 -> Unary Minus1/1

== system Tricopter_Controlled/TriCopter FCS/TriCopter FCS/Flight mode manager and commands generator/Commands generator/Off//Ready ==
  Init comands : Inport
  Gains : Inport  Port=2
  Left_up : Inport  Port=3
  Left_side : Inport  Port=4
  Right_up : Inport  Port=5
  Right_side : Inport  Port=6
  GCS_comm : Inport  Port=7
  Enable : EnablePort  StatesWhenEnabling=reset
  Ground{,1..3} (4 alike) : Ground
  Terminator{,1..5} (6 alike) : Terminator
  Pos_ref(m) : Outport
  Vel_ref_yaw(mps) : Outport  Port=2
  Att_ref(rad) : Outport  Port=3
  omega_b_ref : Outport  Port=4
  wires:
  Gains/1 -> Terminator/1
  Right_up/1 -> Terminator1/1
  Left_up/1 -> Terminator2/1
  Left_side/1 -> Terminator3/1
  Right_side/1 -> Terminator4/1
  GCS_comm/1 -> Terminator5/1
  Ground/1 -> Pos_ref(m)/1
  Ground1/1 -> Att_ref(rad)/1
  Ground2/1 -> Vel_ref_yaw(mps)/1
  Ground3/1 -> omega_b_ref/1

== system Tricopter_Controlled/TriCopter FCS/TriCopter FCS/Flight mode manager and commands generator/Commands generator/Stab ==
  Init comands : Inport
  Gains : Inport  Port=2
  Left_up : Inport  Port=3
  Left_side : Inport  Port=4
  Right_up : Inport  Port=5
  Right_side : Inport  Port=6
  GCS_comm : Inport  Port=7
  Enable : EnablePort  StatesWhenEnabling=reset  ShowOutputPort=on
  Bus Selector : BusSelector  OutputSignals=Vz_yaw_comm,head_comm
  Bus Selector1 : BusSelector  OutputSignals=K_vz,K_phi,K_theta,K_yaw
  Bus Selector2 : BusSelector  OutputSignals=Vel_yaw_z_sp,att_sp
  Divide{1..4} (4 alike) : Product  Inputs=**
  GCS params safemode2 : XXCopter_Control/GCS params safemode
  GCS params safemode3 : XXCopter_Control/GCS params safemode
  Ground{,2..4} (4 alike) : Ground
  Mux : Mux  Inputs=[2,1]
  Mux1 : Mux  Inputs=[2,1]
  Mux2 : Mux  Inputs=3
  Selector : Selector  InputPortWidth=3  Indices=3
  Sum{3,6,8..9} (4 alike) : Sum  Inputs=|++
  Unary Minus : UnaryMinus
  Unary Minus1 : UnaryMinus
  deg2rad1 : Gain  Gain=pi/180
  Pos_ref(m) : Outport
  Vel_ref_yaw(mps) : Outport  Port=2
  Att_ref(rad) : Outport  Port=3
  omega_b_ref : Outport  Port=4
  wires:
  Mux1/1 -> Vel_ref_yaw(mps)/1
  Mux2/1 -> Att_ref(rad)/1
  Mux/1 -> Pos_ref(m)/1
  Ground/1 -> omega_b_ref/1
  GCS_comm/1 -> Bus Selector/1
  Bus Selector/1 -> GCS params safemode2/2  "<Vz_yaw_comm>"
  Bus Selector/2 -> deg2rad1/1  "<head_comm>"
  deg2rad1/1 -> GCS params safemode3/2
  Bus Selector2/1 -> Sum3/1  "<Vel_yaw_z_sp>"
  Gains/1 -> Bus Selector1/1
  Init comands/1 -> Bus Selector2/1
  Sum3/1 -> Sum6/1
  Divide3/1 -> Sum3/2
  Left_up/1 -> Divide3/2
  Ground4/1 -> Mux/1
  GCS params safemode2/1 -> Sum6/2
  Sum6/1 -> Unary Minus/1
  Right_up/1 -> Divide1/1
  Right_side/1 -> Divide2/1
  Sum8/1 -> Sum9/1
  Selector/1 -> Sum8/1
  Bus Selector2/2 -> Selector/1  "<att_sp>"
  Left_side/1 -> Divide4/2
  Divide4/1 -> Sum8/2
  Sum9/1 -> Mux2/3
  GCS params safemode3/1 -> Sum9/2
  Ground2/1 -> Mux1/1
  Unary Minus/1 -> Mux1/2
  Bus Selector1/1 -> Divide3/1  "<K_vz>"
  Bus Selector1/4 -> Divide4/1  "<K_yaw>"
  Bus Selector1/2 -> Divide2/2  "<K_phi>"
  Bus Selector1/3 -> Divide1/2  "<K_theta>"
  Enable/1 -> GCS params safemode3/1, GCS params safemode2/1
  Ground3/1 -> Mux/2
  Divide2/1 -> Mux2/1
  Divide1/1 -> Unary Minus1/1
  Unary Minus1/1 -> Mux2/2

== system Tricopter_Controlled/TriCopter FCS/TriCopter FCS/Flight mode manager and commands generator/Commands generator/Take off ==
  Init comands : Inport
  Gains : Inport  Port=2
  Left_up : Inport  Port=3
  Left_side : Inport  Port=4
  Right_up : Inport  Port=5
  Right_side : Inport  Port=6
  GCS_comm : Inport  Port=7
  Enable : EnablePort  StatesWhenEnabling=reset  ShowOutputPort=on
  Bus Selector : BusSelector  OutputSignals=K_alt
  Bus Selector1 : BusSelector  OutputSignals=Alt_sp
  Bus Selector2 : BusSelector  OutputSignals=Alt_com
  Divide : Product  Inputs=**
  GCS params safemode : XXCopter_Control/GCS params safemode
  Ground{,1..4} (5 alike) : Ground
  Mux : Mux  Inputs=[2,1]
  Mux1 : Mux  Inputs=[2,1]
  Mux2 : Mux  Inputs=3
  Sum : Sum  Inputs=|++
  Sum1 : Sum  Inputs=|++
  Terminator : Terminator
  Terminator1 : Terminator
  Terminator2 : Terminator
  Unary Minus : UnaryMinus
  Pos_ref(m) : Outport
  Vel_ref_yaw(mps) : Outport  Port=2
  Att_ref(rad) : Outport  Port=3
  omega_b_ref : Outport  Port=4
  wires:
  Mux1/1 -> Vel_ref_yaw(mps)/1
  Mux/1 -> Pos_ref(m)/1
  Mux2/1 -> Att_ref(rad)/1
  Gains/1 -> Bus Selector/1
  Init comands/1 -> Bus Selector1/1
  Unary Minus/1 -> Mux/2
  GCS_comm/1 -> Bus Selector2/1
  Bus Selector1/1 -> Sum/1  "<Alt_sp>"
  Bus Selector/1 -> Divide/1  "<K_alt>"
  Left_up/1 -> Divide/2
  Divide/1 -> Sum/2
  Sum/1 -> Sum1/1
  GCS params safemode/1 -> Sum1/2
  Sum1/1 -> Unary Minus/1
  Right_up/1 -> Terminator/1
  Left_side/1 -> Terminator1/1
  Right_side/1 -> Terminator2/1
  Ground/1 -> omega_b_ref/1
  Ground1/1 -> Mux2/3, Mux2/2, Mux2/1
  Ground2/1 -> Mux1/1
  Ground3/1 -> Mux1/2
  Ground4/1 -> Mux/1
  Enable/1 -> GCS params safemode/1
  Bus Selector2/1 -> GCS params safemode/2  "<Alt_com>"

== system Tricopter_Controlled/TriCopter FCS/TriCopter FCS/Flight mode manager and commands generator/Commands generator/Vel_height_auto ==
  Init comands : Inport
  Gains : Inport  Port=2
  Left_up : Inport  Port=3
  Left_side : Inport  Port=4
  Right_up : Inport  Port=5
  Right_side : Inport  Port=6
  GCS_comm : Inport  Port=7
  Enable : EnablePort  StatesWhenEnabling=reset  ShowOutputPort=on
  Bus Selector : BusSelector  OutputSignals=Vx_yaw_comm,Vy_yaw_comm,Alt_com,head_comm,theta_comm
  Bus Selector1 : BusSelector  OutputSignals=K_vx,K_vy,K_alt,K_yaw
  Bus Selector2 : BusSelector  OutputSignals=Vel_yaw_xy_sp,Alt_sp,att_sp
  Demux : Demux  Outputs=2
  Divide{1..4} (4 alike) : Product  Inputs=**
  GCS params safemode{,1..4} (5 alike) : XXCopter_Control/GCS params safemode
  Ground{,1..3} (4 alike) : Ground
  Mux : Mux  Inputs=[2,1]
  Mux1 : Mux  Inputs=[2,1]
  Mux2 : Mux  Inputs=3
  Mux4 : Mux  Inputs=2
  Selector : Selector  InputPortWidth=3  Indices=3
  Selector1 : Selector  InputPortWidth=3  Indices=2
  Sum1 : Sum  Inputs=++|
  Sum{2..9} (8 alike) : Sum  Inputs=|++
  Unary Minus : UnaryMinus
  deg2rad1 : Gain  Gain=pi/180
  deg2rad2 : Gain  Gain=pi/180
  Pos_ref(m) : Outport
  Vel_ref_yaw(mps) : Outport  Port=2
  Att_ref(rad) : Outport  Port=3
  omega_b_ref : Outport  Port=4
  wires:
  Mux1/1 -> Vel_ref_yaw(mps)/1
  Mux2/1 -> Att_ref(rad)/1
  Unary Minus/1 -> Mux/2
  Ground1/1 -> Mux2/1
  Mux4/1 -> Mux1/1
  Ground3/1 -> Mux1/2
  Ground/1 -> omega_b_ref/1
  Mux/1 -> Pos_ref(m)/1
  Gains/1 -> Bus Selector1/1
  Init comands/1 -> Bus Selector2/1
  GCS_comm/1 -> Bus Selector/1
  Sum4/1 -> Sum5/1
  Divide2/1 -> Sum4/2
  Bus Selector2/2 -> Sum4/1  "<Alt_sp>"
  Bus Selector2/1 -> Demux/1  "<Vel_yaw_xy_sp>"
  Sum1/1 -> Sum2/1
  Demux/1 -> Sum1/2
  Right_up/1 -> Divide1/1
  Divide1/1 -> Sum1/1
  Bus Selector1/1 -> Divide1/2  "<K_vx>"
  Bus Selector/1 -> GCS params safemode/2  "<Vx_yaw_comm>"
  GCS params safemode/1 -> Sum2/2
  Bus Selector/2 -> GCS params safemode1/2  "<Vy_yaw_comm>"
  Bus Selector/3 -> GCS params safemode2/2  "<Alt_com>"
  Bus Selector/4 -> deg2rad1/1  "<head_comm>"
  Bus Selector/5 -> deg2rad2/1  "<theta_comm>"
  GCS params safemode2/1 -> Sum5/2
  Sum5/1 -> Unary Minus/1
  Bus Selector1/3 -> Divide2/2  "<K_alt>"
  Left_up/1 -> Divide2/1
  Sum3/1 -> Sum6/1
  Divide3/1 -> Sum3/2
  Right_side/1 -> Divide3/1
  Bus Selector1/2 -> Divide3/2  "<K_vy>"
  Demux/2 -> Sum3/1
  Sum2/1 -> Mux4/1
  Sum6/1 -> Mux4/2
  GCS params safemode1/1 -> Sum6/2
  Sum7/1 -> Sum8/1
  Selector/1 -> Sum7/1
  Left_side/1 -> Divide4/2
  Bus Selector2/3 -> Selector/1, Selector1/1  "<att_sp>"
  Bus Selector1/4 -> Divide4/1  "<K_yaw>"
  Sum8/1 -> Mux2/3
  Selector1/1 -> Sum9/1
  Sum9/1 -> Mux2/2
  Divide4/1 -> Sum7/2
  GCS params safemode3/1 -> Sum8/2
  GCS params safemode4/1 -> Sum9/2
  Ground2/1 -> Mux/1
  deg2rad1/1 -> GCS params safemode3/2
  deg2rad2/1 -> GCS params safemode4/2
  Enable/1 -> GCS params safemode4/1, GCS params safemode3/1, GCS params safemode2/1, GCS params safemode1/1, GCS params safemode/1

== system Tricopter_Controlled/TriCopter FCS/TriCopter FCS/Flight mode manager and commands generator/Commands generator/Vell_auto ==
  Init comands : Inport
  Gains : Inport  Port=2
  Left_up : Inport  Port=3
  Left_side : Inport  Port=4
  Right_up : Inport  Port=5
  Right_side : Inport  Port=6
  GCS_comm : Inport  Port=7
  Enable : EnablePort  StatesWhenEnabling=reset  ShowOutputPort=on
  Bus Selector : BusSelector  OutputSignals=Vx_yaw_comm,Vy_yaw_comm,Vz_yaw_comm,head_comm,theta_comm
  Bus Selector1 : BusSelector  OutputSignals=K_vx,K_vy,K_vz,K_yaw
  Bus Selector2 : BusSelector  OutputSignals=Vel_yaw_xy_sp,Vel_yaw_z_sp,att_sp
  Demux : Demux  Outputs=2
  Divide{1..4} (4 alike) : Product  Inputs=**
  GCS params safemode{,1..4} (5 alike) : XXCopter_Control/GCS params safemode
  Ground{,1,4..5} (4 alike) : Ground
  Mux : Mux  Inputs=[2,1]
  Mux1 : Mux  Inputs=[2,1]
  Mux2 : Mux  Inputs=3
  Mux4 : Mux  Inputs=2
  Selector : Selector  InputPortWidth=3  Indices=3
  Selector1 : Selector  InputPortWidth=3  Indices=2
  Sum1 : Sum  Inputs=++|
  Sum{2..9} (8 alike) : Sum  Inputs=|++
  Unary Minus : UnaryMinus
  deg2rad1 : Gain  Gain=pi/180
  deg2rad2 : Gain  Gain=pi/180
  Pos_ref(m) : Outport
  Vel_ref_yaw(mps) : Outport  Port=2
  Att_ref(rad) : Outport  Port=3
  omega_b_ref : Outport  Port=4
  wires:
  Mux1/1 -> Vel_ref_yaw(mps)/1
  Mux2/1 -> Att_ref(rad)/1
  Ground1/1 -> Mux2/1
  Mux/1 -> Pos_ref(m)/1
  GCS_comm/1 -> Bus Selector/1
  Bus Selector/1 -> GCS params safemode/2  "<Vx_yaw_comm>"
  Bus Selector/2 -> GCS params safemode1/2  "<Vy_yaw_comm>"
  Bus Selector/3 -> GCS params safemode2/2  "<Vz_yaw_comm>"
  Bus Selector/4 -> deg2rad1/1  "<head_comm>"
  Bus Selector/5 -> deg2rad2/1  "<theta_comm>"
  Bus Selector2/1 -> Demux/1  "<Vel_yaw_xy_sp>"
  Gains/1 -> Bus Selector1/1
  Init comands/1 -> Bus Selector2/1
  Sum3/1 -> Sum6/1
  Divide3/1 -> Sum3/2
  Left_up/1 -> Divide3/2
  Bus Selector1/3 -> Divide3/1  "<K_vz>"
  Ground5/1 -> Mux/2
  Ground4/1 -> Mux/1
  Bus Selector2/2 -> Sum3/1  "<Vel_yaw_z_sp>"
  GCS params safemode2/1 -> Sum6/2
  Unary Minus/1 -> Mux1/2
  Sum6/1 -> Unary Minus/1
  Sum1/1 -> Sum2/1
  Demux/1 -> Sum1/2
  Right_up/1 -> Divide1/1
  Divide1/1 -> Sum1/1
  Bus Selector1/1 -> Divide1/2  "<K_vx>"
  GCS params safemode/1 -> Sum2/2
  Sum4/1 -> Sum5/1
  Demux/2 -> Sum4/1
  Sum2/1 -> Mux4/2
  GCS params safemode1/1 -> Sum5/2
  Sum5/1 -> Mux4/1
  Divide2/1 -> Sum4/2
  Bus Selector1/2 -> Divide2/2  "<K_vy>"
  Right_side/1 -> Divide2/1
  Mux4/1 -> Mux1/1
  Sum8/1 -> Sum9/1
  Selector/1 -> Sum8/1
  Bus Selector2/3 -> Selector1/1, Selector/1  "<att_sp>"
  Left_side/1 -> Divide4/2
  Divide4/1 -> Sum8/2
  Sum9/1 -> Mux2/3
  GCS params safemode3/1 -> Sum9/2
  Bus Selector1/4 -> Divide4/1  "<K_yaw>"
  Sum7/1 -> Mux2/2
  GCS params safemode4/1 -> Sum7/2
  Selector1/1 -> Sum7/1
  deg2rad1/1 -> GCS params safemode3/2
  deg2rad2/1 -> GCS params safemode4/2
  Enable/1 -> GCS params safemode4/1, GCS params safemode3/1, GCS params safemode2/1, GCS params safemode1/1, GCS params safemode/1
  Ground/1 -> omega_b_ref/1

== system Tricopter_Controlled/TriCopter FCS/TriCopter FCS/Flight mode manager and commands generator/Commands generator/commnads_gen_logic ==
  flight_mode : Inport
  All_meas : Inport  Port=2
  Enable : EnablePort  StatesWhenEnabling=reset
  Bus Creator : BusCreator  Inputs=12  OutDataTypeStr=Bus: manual_gains
  Bus Creator1 : BusCreator  Inputs=6  OutDataTypeStr=Bus: commander_sp
  Bus Selector1 : BusSelector  OutputSignals=Meas.Pos_meas_m,Params.V_yaw,Meas.Eulr_meas_rad
  Signal Conversion : SignalConversion
  Signal Conversion1 : SignalConversion
  commands_generator : MATLAB Function  TreatAsAtomicUnit=on
  set_points : Outport
  gains : Outport  Port=2
  wires:
  All_meas/1 -> Bus Selector1/1
  Bus Selector1/1 -> commands_generator/2(Xe)  "<Pos_meas_m>"
  Bus Selector1/2 -> commands_generator/3(V_yaw)  "<V_yaw>"
  Bus Selector1/3 -> commands_generator/4(Euler)  "<Eulr_meas_rad>"
  commands_generator/1(Loc_XY_sp) -> Bus Creator1/1  "Loc_XY_sp"
  commands_generator/2(Alt_sp) -> Bus Creator1/2  "Alt_sp"
  commands_generator/3(Vel_yaw_xy_sp) -> Bus Creator1/3  "Vel_yaw_xy_sp"
  commands_generator/4(Vel_yaw_z_sp) -> Bus Creator1/4  "Vel_yaw_z_sp"
  commands_generator/5(att_sp) -> Bus Creator1/5  "att_sp"
  commands_generator/16(K_p) -> Bus Creator/10  "K_p"
  commands_generator/17(K_q) -> Bus Creator/11  "K_q"
  commands_generator/18(K_r) -> Bus Creator/12  "K_r"
  Bus Creator/1 -> Signal Conversion1/1  "manual_gains"
  flight_mode/1 -> commands_generator/1(flight_mode)
  commands_generator/6(omega_b_sp) -> Bus Creator1/6  "omega_b_sp"
  commands_generator/7(K_alt) -> Bus Creator/1  "K_alt"
  commands_generator/8(K_x) -> Bus Creator/2  "K_x"
  commands_generator/9(K_y) -> Bus Creator/3  "K_y"
  commands_generator/15(K_yaw) -> Bus Creator/9  "K_yaw"
  commands_generator/10(K_vx) -> Bus Creator/4  "K_vx"
  commands_generator/11(K_vy) -> Bus Creator/5  "K_vy"
  commands_generator/12(K_vz) -> Bus Creator/6  "K_vz"
  commands_generator/13(K_phi) -> Bus Creator/7  "K_phi"
  commands_generator/14(K_theta) -> Bus Creator/8  "K_theta"
  Bus Creator1/1 -> Signal Conversion/1  "commander_sp"
  Signal Conversion/1 -> set_points/1
  Signal Conversion1/1 -> gains/1

== system Tricopter_Controlled/TriCopter FCS/Simulink to px4 input/Flat Earth to LLA/ne to lat//long/LongLat_offset /Find Radian//Distance  ==
  note: R
  mu : Inport
  Constant{,2..3,5..6} (5 alike) : Constant
  Constant1 : Constant  Value=6378137
  Constant4 : Constant  Value=1/298.257223563
  Product1 : Product  Inputs=*/  RndMeth=Zero
  Product2 : Product  RndMeth=Zero
  Product3 : Product  Inputs=**/  RndMeth=Zero
  Product4 : Product  RndMeth=Zero
  Product5 : Product  RndMeth=Zero
  Product6 : Product  Inputs=4  RndMeth=Zero
  Sum : Sum  Inputs=-+
  Sum1 : Sum  Inputs=|+-
  Sum2 : Sum  Inputs=|+-
  Sum3 : Sum  Inputs=|+-
  Trigonometric Function : Trigonometry  Operator=cos
  Trigonometric Function1 : Trigonometry  Operator=atan2
  Trigonometric Function2 : Trigonometry  Operator=atan2
  Trigonometric Function3 : Trigonometry
  deg2rad : Gain  Gain=pi/180  SaturateOnIntegerOverflow=on  OutDataTypeStr=Inherit: Same as input  ParamDataTypeStr=Inherit: Same as input
  f : Constant
  sqrt : Sqrt  AlgorithmType=Newton-Raphson  SaturateOnIntegerOverflow=on
  sqrt1 : Sqrt  AlgorithmType=Newton-Raphson  SaturateOnIntegerOverflow=on
  dNorth : Outport
  dEast : Outport  Port=2
  wires:
  Trigonometric Function2/1 -> dEast/1
  Trigonometric Function1/1 -> dNorth/1
  Constant3/1 -> Trigonometric Function2/1
  Constant2/1 -> Trigonometric Function1/1
  Product4/1 -> Trigonometric Function2/2
  mu/1 -> deg2rad/1
  Trigonometric Function/1 -> Product4/2
  Product3/1 -> Trigonometric Function1/2  "Rm"
  Sum1/1 -> Product3/2
  Product1/1 -> Product4/1, Product3/1  "Rn"
  Constant/1 -> Sum1/1
  Product2/1 -> Sum1/2
  Constant1/1 -> Product1/1
  sqrt/1 -> Product1/2
  Sum3/1 -> Product3/3, sqrt/1
  f/1 -> Sum/2
  Constant4/1 -> Sum/1
  Sum/1 -> Product5/1, Product5/2
  Product5/1 -> Sum2/2
  Constant5/1 -> Sum2/1
  Sum2/1 -> sqrt1/1
  deg2rad/1 -> Trigonometric Function3/1, Trigonometric Function/1
  Trigonometric Function3/1 -> Product6/4, Product6/3
  sqrt1/1 -> Product6/1, Product6/2, Product2/2, Product2/1
  Product6/1 -> Sum3/2
  Constant6/1 -> Sum3/1
